simulink model "BANSHEE_v2"  (Simulink 8.1)
settings: Solver=ode1  StartTime=0.0  StopTime=inf  FixedStep=Ts  MaxStep=1e-3  RelTol=1e-3
model workspace (MAT data in the model file):
  op_snapshot1 : opcond.OperatingPoint (value not decoded)
PostLoadFcn:
  | BANSHEE_init;
InitFcn:
  | BANSHEE_init;
values from neighbouring files (symbols this model uses):
  F1 = xlsread('F1_relay_banshee.xlsx')    [relay_settings_init.m]
  F2 = xlsread('F2_relay_banshee.xlsx')    [relay_settings_init.m]
  F3 = xlsread('F3_relay_banshee.xlsx')    [relay_settings_init.m]
  Ts = 100E-6    (= 0.0001)    [BANSHEE_init.m]
undefined symbols (not defined in the file or in its folder): cable_spec, fdesignblkfcn, Feeder1_lib, Feeder2_lib, Feeder3_lib, gcbh, generic_ethernet_cb, Left, relay_housing_lib, SM_UtilityService, SS_F1_RELAY_HOUSING, SS_F2_RELAY_HOUSING, SS_F3_RELAY_HOUSING, SS_Feeder1, SS_Feeder2, SS_Feeder3, type, utility_service_lib, V
libraries: breaker_lib x51, rtio_generic_modbus x43, relay_modbus_lib x42, cables_lib x34, artemis x24, transformer_lib x24, Load_lib x18, simulink x16, ssn_lib x16, rtlab x15, rtio_opalrt_common x15, PQFV_lib x8
(part 1 of 5)
settings Model: ARTEMISmethode_block_infos=$$__separator__$$BANSHEE_v2/ARTEMIS Guide$$__separator__$$  Creator=RE25624  LastModifiedBy=re25624  BufferReuse=off
settings SolverCC: ZeroCrossAlgorithm=Adaptive
settings DataIOCC: ExternalInput=getinputstruct(op_snapshot1)  InitialState=getstatestruct(op_snapshot1)  LimitDataPoints=off  MaxDataPoints=90060  SignalLoggingSaveFormat=Dataset  SaveOutput=off  SignalLogging=off  DSMLogging=off  SaveTime=off  OutputSaveName=result
settings OptimizationCC: BlockReduction=off  OptimizeBlockIOStorage=off  BufferReuse=off  ExpressionFolding=off  LocalBlockOutputs=off
settings DebuggingCC: MaxConsecutiveZCsMsg=warning  IgnoredZcDiagnostic=none  SolverPrmCheckMsg=none  MultiTaskRateTransMsg=warning  FcnCallInpInsideContextMsg=EnableAllAsWarning  FrameProcessingCompatibilityMsg=error  ModelReferenceExtraNoncontSigs=warning  StrictBusMsg=None
settings ModelReferenceCC: UpdateModelReferenceTargets=IfOutOfDate
settings SFSimCC: SFSimEcho=off
settings GRTTargetCC: CodeReplacementLibrary=C89/C90 (ANSI)

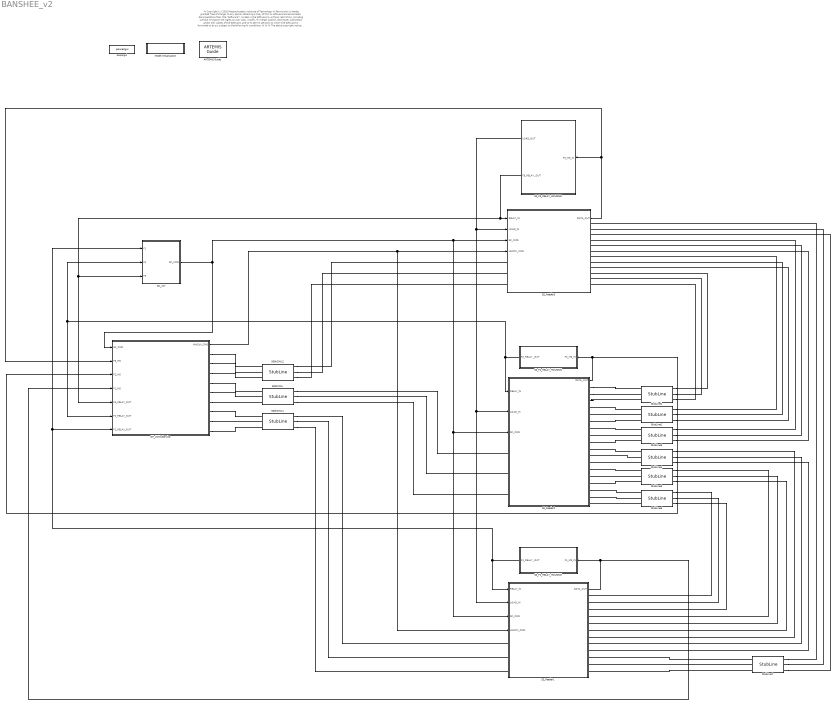
== system BANSHEE_v2 ==
  note: % Copyright (c) 2016 Massachusetts Institute of Technology
      | % Permission is hereby granted, free of charge, to any person obtaining a copy of this
      | % software and associated documentation files (the "Software"), to deal in the Software
      | % without restriction, including without limitation the rights to use, copy, modify,
      | % merge, publish, distribute, sublicense, and/or sell copies of the Software, and to
      | % permit persons to whom the Software is furnished to do so, subject to the following
      | % conditions:
      | %
      | %
      | % The above copyright notice and this permission notice shall be included in
      | % all copies or substantial portions of the Software.
      | %
      | % THE SOFTWARE IS PROVIDED "AS IS", WITHOUT WARRANTY OF ANY KIND, EXPRESS OR IMPLIED,
      | % INCLUDING BUT NOT LIMITED TO THE WARRANTIES OF MERCHANTABILITY, FITNESS FOR A
      | % PARTICULAR PURPOSE AND NONINFRINGEMENT. IN NO EVENT SHALL THE AUTHORS OR COPYRIGHT
      | % HOLDERS BE LIABLE FOR ANY CLAIM, DAMAGES OR OTHER LIABILITY, WHETHER IN AN ACTION
      | % OF CONTRACT, TORT OR OTHERWISE, ARISING FROM, OUT OF OR IN CONNECTION WITH THE
      | % SOFTWARE OR THE USE OR OTHER DEALINGS IN THE SOFTWARE.
      | %
      | %
      | %%
  500kCMIL : artemis/ARTEMIS/StubLine  Phases=3  pu=off  L=10000 * 9.43453e-08 / 1  Lpu=0.08  R=10000 * 2.28409e-5 / 1  Rpu=0.002  S_base=450e6/3  V_base=230e3/sqrt(3)  F_base=60  Ts=Ts
  500kCMIL1 : artemis/ARTEMIS/StubLine  Phases=3  pu=off  L=10000 * 9.43453e-08 / 1  Lpu=0.08  R=10000 * 2.28409e-5 / 1  Rpu=0.002  S_base=450e6/3  V_base=230e3/sqrt(3)  F_base=60  Ts=Ts
  500kCMIL2 : artemis/ARTEMIS/StubLine  Phases=3  pu=off  L=10000 * 9.43453e-08 / 1  Lpu=0.08  R=10000 * 2.28409e-5 / 1  Rpu=0.002  S_base=450e6/3  V_base=230e3/sqrt(3)  F_base=60  Ts=Ts
  ARTEMIS Guide : artemis/ARTEMIS/ARTEMIS Guide  Tag=FTSSmethode_opal_4hx0r99  Description=5.0_z1  lock=on  Ts=Ts  opt=art5  dyna=off  nb_perm=4  RT_fullcomp=off  ssn=on  ssn_itvc=off  ssn_ivic=off  ssn_ext=off  ssn_solver=Art5 with Backward Euler nodal interface  ssn_impulse=off  ssn_quasimpulse=off  ssn_impulse_loop=5  paraExtinctionThy=off  Thy_Impulse=on  dtc=Off  dtc_opt=normal  ao=on  simtype=off  ct_mac=off  lin_mov=off  lsp=[0.001 2]  spike_skip=Disabled  dtc_extra=1  dtc_sws=normal  dtc_pied=0.5  SPSRulesBlock=SPSRules  tre=on  ctmm=off  LF=off  dpl_type=ARTEMiS DPL  rlc_type=off  custom_type=off  para=on  ssn_ImpulseLoopBlockedStateUpdate=5  ssn_mov_iter_number=5  ssn_switch_iter_number=5
  Model Initialization : Subsystem  AncestorBlock=artemis/Tools /Misc/Model Initialization  mask(Model Functions){InitFcnX=BANSHEE_init;, prel=off, posl=on, inif=on, strf=off}
      mask prompts: InitFcnX "Initialisation"; prel "Preload Function"; posl "PostLoad Function"; inif "InitFcn"; strf "StartFcn"
      mask init:
      | currentBlock = gcb;
      | root = bdroot(currentBlock);
      | 
      | if ~strcmp(get_param(root,'BlockDiagramType'),'library')
      |     if prel==1
      |         set_param(root, 'PreLoadFcn', InitFcnX);
      |     else
      |         set_param(root, 'PreLoadFcn', '');
      |     end
      |     if inif==1
      |         set_param(root, 'InitFcn', InitFcnX);
      |     else
      |         set_param(root, 'InitFcn', '');
      |     end
      |     if strf==1
      |         set_param(root, 'StartFcn', InitFcnX);
      |     else
      |         set_param(root, 'StartFcn', '');
      |     end
      |     if posl==1
      |         set_param(root, 'PostLoadFcn', InitFcnX);
      |     else
      |         set_param(root, 'PostLoadFcn', '');
      |     end
      | end
      | 
      | pos = get_param(currentBlock, 'Position');
      | width = pos(3) - pos(1); height = pos(4) - pos(2);
      | txt = [ upper(root) '\n' '- InitFcn. . . . . '  get_param(root, 'InitFcn') ];
      settings: CopyFcn=set_param(gcb,'LinkStatus','inactive')
      mask Display: text(5, height*0.5, txt, 'horizontalAlignment', 'left', 'verticalAlignment', 'middle') ;
  SC_ctrl : Subsystem
  SM_UtilityService : Subsystem  AncestorBlock=utility_service_lib/SM_UtilityService
  SS_F1_RELAY_HOUSING : Subsystem  AncestorBlock=relay_housing_lib/SS_F1_RELAY_HOUSING
  SS_F2_RELAY_HOUSING : Subsystem  AncestorBlock=relay_housing_lib/SS_F2_RELAY_HOUSING
  SS_F3_RELAY_HOUSING : Subsystem  AncestorBlock=relay_housing_lib/SS_F3_RELAY_HOUSING
  SS_Feeder1 : Subsystem  AncestorBlock=Feeder1_lib/SS_Feeder1
  SS_Feeder2 : Subsystem  AncestorBlock=Feeder2_lib/SS_Feeder2
  SS_Feeder3 : Subsystem  AncestorBlock=Feeder3_lib/SS_Feeder3
  StubLine1 : artemis/ARTEMIS/StubLine  Phases=3  pu=off  L=1500 * 9.43453e-08 / 2  Lpu=0.08  R=1500 * 2.28409e-5 / 2  Rpu=0.002  S_base=450e6/3  V_base=230e3/sqrt(3)  F_base=60  Ts=Ts
  StubLine2 : artemis/ARTEMIS/StubLine  Phases=3  pu=off  L=1500 * 9.43453e-08 / 2  Lpu=0.08  R=1500 * 2.28409e-5 / 2  Rpu=0.002  S_base=450e6/3  V_base=230e3/sqrt(3)  F_base=60  Ts=Ts
  StubLine3 : artemis/ARTEMIS/StubLine  Phases=3  pu=off  L=1500 * 9.43453e-08 / 2  Lpu=0.08  R=1500 * 2.28409e-5 / 2  Rpu=0.002  S_base=450e6/3  V_base=230e3/sqrt(3)  F_base=60  Ts=Ts
  StubLine4 : artemis/ARTEMIS/StubLine  Phases=3  pu=off  L=1000 * 9.43453e-08 / 2  Lpu=0.08  R=1000 * 2.28409e-5 / 2  Rpu=0.002  S_base=450e6/3  V_base=230e3/sqrt(3)  F_base=60  Ts=Ts
  StubLine5 : artemis/ARTEMIS/StubLine  Phases=3  pu=off  L=2000 * 9.43453e-08 / 2  Lpu=0.08  R=2000 * 2.28409e-5 / 2  Rpu=0.002  S_base=450e6/3  V_base=230e3/sqrt(3)  F_base=60  Ts=Ts
  StubLine6 : artemis/ARTEMIS/StubLine  Phases=3  pu=off  L=3000 * 9.43453e-08 / 1  Lpu=0.08  R=3000 * 2.28409e-5 / 1  Rpu=0.002  S_base=450e6/3  V_base=230e3/sqrt(3)  F_base=60  Ts=Ts
  StubLine7 : artemis/ARTEMIS/StubLine  Phases=3  pu=off  L=2000 * 9.43453e-08 / 2  Lpu=0.08  R=2000 * 2.28409e-5 / 2  Rpu=0.002  S_base=450e6/3  V_base=230e3/sqrt(3)  F_base=60  Ts=Ts
  powergui : powerlib/powergui  Priority=2  SimulationMode=Discrete  SolverType=Tustin  SampleTime=Ts  frequency=60  SPID=off  DisableSnubberDevices=off  DisableRonSwitches=off  DisableVfSwitches=off  SwTol=0  Interpol=off  DisplayEquations=off  frequencyindice=0  Pbase=100e6  ErrMax=1e-4  Iterations=50  UnitsV=kV  UnitsW=MW  FunctionMessages=off  echomessages=off  HookPort=off  EnableUseOfTLC=off  x0status=blocks  RestoreLinks=warning  ResistiveCurrentMeasurement=off  Frange=logspace(0,3,50)  Ylog=off  Xlog=off  ShowGrid=off  save=off  variable=ZData  structure=0  ZoomFFT=on  StartTime=0.0  cycles=2  DisplayStyle=off  fundamental=60  FreqAxis=off  MaxFrequency=1000  frequencyindicesteady=1  RmsSteady=1  display=off  Ts=0  methode=off
  wires:
  SS_Feeder3/1(DATA_OUT) -> SM_UtilityService/2(F3_MS), SS_F3_RELAY_HOUSING/1(F3_MS_IN)
  SS_F3_RELAY_HOUSING/2(F3_RELAY _OUT) -> SM_UtilityService/5(F3_RELAY_OUT), SC_ctrl/3(F3), SS_Feeder3/1(RELAY_IN)
  SS_F1_RELAY_HOUSING/1(F1_RELAY _OUT) -> SS_Feeder1/1(RELAY_IN), SC_ctrl/1(F1), SM_UtilityService/7(F1_RELAY_OUT)
  SS_F2_RELAY_HOUSING/1(F2_RELAY _OUT) -> SC_ctrl/2(F2), SM_UtilityService/6(F2_RELAY_OUT), SS_Feeder2/1(RELAY_IN)
  SS_Feeder1/1(DATA_OUT) -> SM_UtilityService/4(F1_MS), SS_F1_RELAY_HOUSING/1(F1_MS_IN)
  SS_Feeder2/1(DATA_OUT) -> SM_UtilityService/3(F2_MS), SS_F2_RELAY_HOUSING/1(F2_MS_IN)
  SC_ctrl/1(SC_CMD) -> SM_UtilityService/1(SC_CMD), SS_Feeder1/3(SC_CMD), SS_Feeder2/3(SC_CMD), SS_Feeder3/3(SC_CMD)
  SS_F3_RELAY_HOUSING/1(LOAD_OUT) -> SS_Feeder3/2(LOAD_IN), SS_Feeder1/2(LOAD_IN), SS_Feeder2/2(LOAD_IN)
  SM_UtilityService/1(HWCtrl_CMD) -> SS_Feeder1/4(HWCtrl_CMD), SS_Feeder3/4(HWCtrl_CMD)
  connections:
  SS_Feeder2/RConn2 -- StubLine1/LConn2
  SS_Feeder2/RConn1 -- StubLine1/LConn1
  SS_Feeder2/RConn3 -- StubLine1/LConn3
  StubLine2/LConn2 -- SS_Feeder2/RConn5
  StubLine2/LConn3 -- SS_Feeder2/RConn6
  StubLine2/LConn1 -- SS_Feeder2/RConn4
  StubLine3/LConn2 -- SS_Feeder2/RConn8
  StubLine3/LConn1 -- SS_Feeder2/RConn7
  StubLine3/LConn3 -- SS_Feeder2/RConn9
  StubLine4/LConn3 -- SS_Feeder2/RConn12
  StubLine4/LConn2 -- SS_Feeder2/RConn11
  StubLine4/LConn1 -- SS_Feeder2/RConn10
  StubLine7/LConn3 -- SS_Feeder1/RConn12
  StubLine7/LConn2 -- SS_Feeder1/RConn11
  StubLine7/LConn1 -- SS_Feeder1/RConn10
  StubLine5/LConn2 -- SS_Feeder2/RConn14
  StubLine5/LConn1 -- SS_Feeder2/RConn13
  StubLine5/LConn3 -- SS_Feeder2/RConn15
  StubLine6/LConn3 -- SS_Feeder2/RConn18
  StubLine6/LConn2 -- SS_Feeder2/RConn17
  StubLine6/LConn1 -- SS_Feeder2/RConn16
  StubLine6/RConn1 -- SS_Feeder1/RConn1
  StubLine6/RConn2 -- SS_Feeder1/RConn2
  StubLine6/RConn3 -- SS_Feeder1/RConn3
  StubLine5/RConn1 -- SS_Feeder1/RConn4
  StubLine5/RConn2 -- SS_Feeder1/RConn5
  StubLine5/RConn3 -- SS_Feeder1/RConn6
  StubLine4/RConn1 -- SS_Feeder1/RConn7
  StubLine4/RConn2 -- SS_Feeder1/RConn8
  StubLine4/RConn3 -- SS_Feeder1/RConn9
  StubLine3/RConn3 -- SS_Feeder3/RConn6
  StubLine3/RConn2 -- SS_Feeder3/RConn5
  StubLine3/RConn1 -- SS_Feeder3/RConn4
  StubLine2/RConn3 -- SS_Feeder3/RConn9
  StubLine2/RConn2 -- SS_Feeder3/RConn8
  StubLine2/RConn1 -- SS_Feeder3/RConn7
  StubLine1/RConn3 -- SS_Feeder3/RConn12
  StubLine1/RConn2 -- SS_Feeder3/RConn11
  StubLine1/RConn1 -- SS_Feeder3/RConn10
  StubLine7/RConn1 -- SS_Feeder3/RConn1
  StubLine7/RConn2 -- SS_Feeder3/RConn2
  StubLine7/RConn3 -- SS_Feeder3/RConn3
  500kCMIL2/RConn3 -- SS_Feeder3/LConn3
  500kCMIL2/RConn2 -- SS_Feeder3/LConn2
  500kCMIL2/RConn1 -- SS_Feeder3/LConn1
  500kCMIL/RConn1 -- SS_Feeder2/LConn1
  500kCMIL/RConn2 -- SS_Feeder2/LConn2
  500kCMIL/RConn3 -- SS_Feeder2/LConn3
  500kCMIL1/RConn1 -- SS_Feeder1/LConn1
  500kCMIL1/RConn2 -- SS_Feeder1/LConn2
  500kCMIL1/RConn3 -- SS_Feeder1/LConn3
  SM_UtilityService/RConn1 -- 500kCMIL2/LConn1
  SM_UtilityService/RConn2 -- 500kCMIL2/LConn2
  SM_UtilityService/RConn3 -- 500kCMIL2/LConn3
  SM_UtilityService/RConn4 -- 500kCMIL/LConn1
  SM_UtilityService/RConn5 -- 500kCMIL/LConn2
  SM_UtilityService/RConn6 -- 500kCMIL/LConn3
  SM_UtilityService/RConn7 -- 500kCMIL1/LConn1
  SM_UtilityService/RConn8 -- 500kCMIL1/LConn2
  SM_UtilityService/RConn9 -- 500kCMIL1/LConn3

== system BANSHEE_v2/Model Initialization ==

== system BANSHEE_v2/SC_ctrl ==
  note: % Copyright (c) 2016 Massachusetts Institute of Technology
      | % Permission is hereby granted, free of charge, to any person obtaining a copy of this
      | % software and associated documentation files (the "Software"), to deal in the Software
      | % without restriction, including without limitation the rights to use, copy, modify,
      | % merge, publish, distribute, sublicense, and/or sell copies of the Software, and to
      | % permit persons to whom the Software is furnished to do so, subject to the following
      | % conditions:
      | %
      | %
      | % The above copyright notice and this permission notice shall be included in
      | % all copies or substantial portions of the Software.
      | %
      | % THE SOFTWARE IS PROVIDED "AS IS", WITHOUT WARRANTY OF ANY KIND, EXPRESS OR IMPLIED,
      | % INCLUDING BUT NOT LIMITED TO THE WARRANTIES OF MERCHANTABILITY, FITNESS FOR A
      | % PARTICULAR PURPOSE AND NONINFRINGEMENT. IN NO EVENT SHALL THE AUTHORS OR COPYRIGHT
      | % HOLDERS BE LIABLE FOR ANY CLAIM, DAMAGES OR OTHER LIABILITY, WHETHER IN AN ACTION
      | % OF CONTRACT, TORT OR OTHERWISE, ARISING FROM, OUT OF OR IN CONNECTION WITH THE
      | % SOFTWARE OR THE USE OR OTHER DEALINGS IN THE SOFTWARE.
      | %
      | %
      | %%
  note: The 'Overruns' value should remain at 0.
      | The 'Ttotal' value should be equal to the
      | model Fixed-Step size.
  F1 : Inport
  F2 : Inport  Port=2
  F3 : Inport  Port=3
  1: connect motor 0: disconnect motor : Constant  Value=0
  Bus Creator1 : BusCreator
  Gen_3.5MVA : Subsystem
  OpComm : rtlab/OpComm  nbport=3  groupe_acq=1  subsys_rate=0  st=0  Synchronization=on  Interpolation=on  Threshold=1.0  Missed_Data=off  Sim_Time=off  Samples=off  dynSigOut=off  from_console=0  warning_done=off  writeOpCommFile=off  Offset=off
  Overall : Subsystem
  Status : Subsystem
  Woodward : Subsystem
  opElectricFaultSelector : artemis/Tools /POW faults/opElectricFaultSelector  phase_a=on  phase_b=on  phase_c=on  gnd_fault=on  Tacq=1  Tst=[0.1 0 10]  enable_POW=off  angle_POW=[15 0 10]  Tdr="[0.5 0  10]"  fault_location_menu=No fault  T_init=2
  SC_CMD : Outport
  wires:
  F1/1 -> OpComm/1
  F2/1 -> OpComm/2
  F3/1 -> OpComm/3
  OpComm/1 -> Overall/1(F1), Status/1(F1)
  OpComm/2 -> Status/2(F2), Overall/2(F2)
  OpComm/3 -> Status/3(F3), Overall/3(F3)
  opElectricFaultSelector/1 -> [fault_cmd]
  Bus Creator1/1 -> SC_CMD/1
  1: connect motor 0: disconnect motor/1 -> Bus Creator1/2  "motor_signals"
  [IO_ctrl] -> Bus Creator1/3  "IO ctrl"
  Gen_3.5MVA/1(S) -> Bus Creator1/1  "NGCHP_ManualCtrl"
  Woodward/1(IOctrl) -> [IO_ctrl]
  [fault_cmd] -> Bus Creator1/4  "fault_cmd"

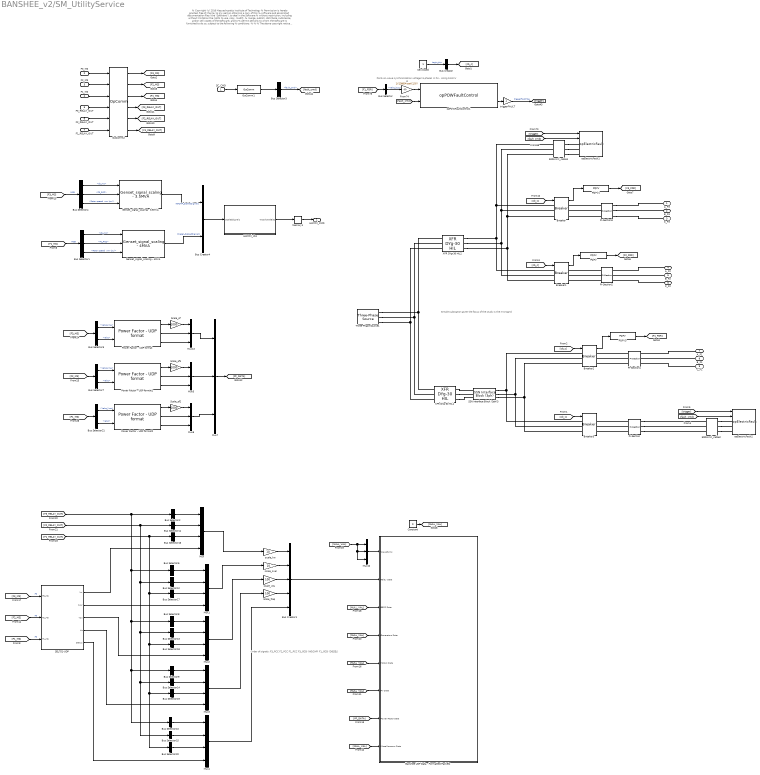
== system BANSHEE_v2/SM_UtilityService ==
  note: Simple substation given the focus of the study is the microgrid
  note: % Copyright (c) 2016 Massachusetts Institute of Technology
      | % Permission is hereby granted, free of charge, to any person obtaining a copy of this
      | % software and associated documentation files (the "Software"), to deal in the Software
      | % without restriction, including without limitation the rights to use, copy, modify,
      | % merge, publish, distribute, sublicense, and/or sell copies of the Software, and to
      | % permit persons to whom the Software is furnished to do so, subject to the following
      | % conditions:
      | %
      | %
      | % The above copyright notice and this permission notice shall be included in
      | % all copies or substantial portions of the Software.
      | %
      | % THE SOFTWARE IS PROVIDED "AS IS", WITHOUT WARRANTY OF ANY KIND, EXPRESS OR IMPLIED,
      | % INCLUDING BUT NOT LIMITED TO THE WARRANTIES OF MERCHANTABILITY, FITNESS FOR A
      | % PARTICULAR PURPOSE AND NONINFRINGEMENT. IN NO EVENT SHALL THE AUTHORS OR COPYRIGHT
      | % HOLDERS BE LIABLE FOR ANY CLAIM, DAMAGES OR OTHER LIABILITY, WHETHER IN AN ACTION
      | % OF CONTRACT, TORT OR OTHERWISE, ARISING FROM, OUT OF OR IN CONNECTION WITH THE
      | % SOFTWARE OR THE USE OR OTHER DEALINGS IN THE SOFTWARE.
      | %
      | %
      | %%
  note: Point-on-wave synchronisation voltage (3-phase) in PU - Using 13.8 kV
  note: Order of signals:
      | F3_PCC
      | F2_PCC
      | F1_PCC
      | F3_GCB (NG/CHP)
      | F1_GCB (DIESEL)
  SC_CMD : Inport
  F3_MS : Inport  Port=2
  F2_MS : Inport  Port=3
  F1_MS : Inport  Port=4
  F3_RELAY_OUT : Inport  Port=5
  F2_RELAY_OUT : Inport  Port=6
  F1_RELAY_OUT : Inport  Port=7
  500kcmil_cable1 : cables_lib/500kcmil_cable  length=1  par_sets=1
  500kcmil_cable2 : cables_lib/500kcmil_cable  length=1  par_sets=1
  Banshee UDP Data - Formatted Packets : Subsystem  mask(UDP Data Block){ProfileID=2, NumOfWaveforms=[0, 0, 0], NumOfRelays=[47, [10, 10, 100, 100]], NumOfBatteries=0, NumOfGensets=0, NumOfMotors=0, NumOfPVs=0, NumOfPF=[3, [1000, 1000, 1000]], NumOfMiscellaneousDataScales=0, NumOfMiscellaneousDataSignalsScales=0}
      mask prompts: ProfileID "Profile ID"; NumOfWaveforms "Waveform Data"; NumOfRelays "Relay Data"; NumOfBatteries "# of Batteries"; NumOfGensets "# of Gensets"; NumOfMotors "# of Motors"; NumOfPVs "# of PVs"; NumOfPF "Power Factor Data"; NumOfMiscellaneousDataScales "Misc. Data - No. of Scale Factors"; NumOfMiscellaneousDataSignalsScales "Misc. - No. Signals and Scale Values"
      mask help:
      | * All signal scaling should be external to this block
      |
      | Profile ID: (1-Sheriff, 2-Banshee, 3-Canary, 4-Siren)
      |
      | Waveforms Data: No. of per phase waveforms sent at 5Hz rate, point per waveforms [dt=80us, 208; dt=100us, 166], and scaling factor.
      | -Input format: [No. of waveforms, No. of datapoints, scale]
      | -Ex. for Canary:[3, 166, 100]
      |
      | Relay Data: No. of relays feeding packet data to breakers in display - mapped/indexed in ascending order
      | -Packet order: Active power(kW), reactive power(kVAR), voltage(per-unit), frequency (Hz), breaker status (1:closed, 0:open)
      | -Input format: [No. of Relays, [scale_kW, scale_kVAR, scale_Vpu, scale_Hz]]
      | -Ex. for Canary:[4, [10, 10, 100, 100]]
      |
      | No. of Batteries: TBD
      | -Ex. for Canary: [0]
      | No. of Generators: TBD
      | -Ex. for Canary: [0]
      |
      | Motors Data: No. of motors monitored in the system. Currently, only looking at motor on/off state.
      | -Input format: [No. of motors]
      | -Ex. for Canary: [1]
      |
      | No. of PV: TBD
      | -Ex. for Canary: [0]
      |
      | Power Factor Data: No. of power factors to be displayed in the system, and corresponding scale values.
      | -Packet order: power factor, import/export, lagging/leading
      | -Input format: [No. of Power Factors, [scale_pf]]
      | -Ex. for Canary:[1, [1000]]
      |
      | Misc. Data - No. of Scale factor: NUmber of scale factors to be applied to each signal-set.
      | -Ex. for Canary: [3]
      |
      | Misc. Data - No. of Signals and Scale Values: Size of signal set and scale value to be applied to the signal-set.
      | -Ex. for Canary: [[1, 1000], [6, 100], [3, 10]]
  Breaker{,1..3} (4 alike) : breaker_lib/Breaker  Ts=Ts  mech_delay=cb_mech_delay
  Bus Creator : BusCreator  Inputs=1
  Bus Creator1 : BusCreator  Inputs=5
  Bus Creator4 : BusCreator  Inputs=2
  Bus Selector : BusSelector  OutputSignals=cb_ms.Vabc_bus
  Bus Selector1 : BusSelector  OutputSignals="DIESEL_DATA.DIESEL_GCB.cb_ms,CB_DATA.F1_PCC,DIESEL_DATA.Gen2_meas.w.w.Rotor speed  wm (pu)"
  Bus Selector10 : BusSelector  OutputSignals=F3_CB_1.m.status,F3_CB_2.m.status,F3_CB_3.m.status,F3_CB_4.m.status,F3_CB_5.m.status,F3_CB_6.m.status,F3_CB_7.m.status,F3_CB_8.m.status,F3_CB_9.m.status  OutputAsBus=on
  Bus Selector11 : BusSelector  OutputSignals=F2_CB_1.m.kw,F2_CB_2.m.kw,F2_CB_3.m.kw,F2_CB_4.m.kw,F2_CB_5.m.kw,F2_CB_6.m.kw,F2_CB_7.m.kw,F2_CB_8.m.kw,F2_CB_9.m.kw,F2_CB_10.m.kw,F2_CB_11.m.kw,F2_CB_12.m.kw,F2_CB_13.m.kw,F2_CB_14.m.kw,F2_CB_15.m.kw,F2_CB_16.m.kw,F2_CB_17.m.kw,F2_CB_18.m.kw,F2_CB_19.m.kw  OutputAsBus=on
  Bus Selector12 : BusSelector  OutputSignals=F2_CB_1.m.kvar,F2_CB_2.m.kvar,F2_CB_3.m.kvar,F2_CB_4.m.kvar,F2_CB_5.m.kvar,F2_CB_6.m.kvar,F2_CB_7.m.kvar,F2_CB_8.m.kvar,F2_CB_9.m.kvar,F2_CB_10.m.kvar,F2_CB_11.m.kvar,F2_CB_12.m.kvar,F2_CB_13.m.kvar,F2_CB_14.m.kvar,F2_CB_15.m.kvar,F2_CB_16.m.kvar,F2_CB_17.m.kvar,F2_CB_18.m.kvar,F2_CB_19.m.kvar  OutputAsBus=on
  Bus Selector13 : BusSelector  OutputSignals=F2_CB_1.m.Vpu,F2_CB_2.m.Vpu,F2_CB_3.m.Vpu,F2_CB_4.m.Vpu,F2_CB_5.m.Vpu,F2_CB_6.m.Vpu,F2_CB_7.m.Vpu,F2_CB_8.m.Vpu,F2_CB_9.m.Vpu,F2_CB_10.m.Vpu,F2_CB_11.m.Vpu,F2_CB_12.m.Vpu,F2_CB_13.m.Vpu,F2_CB_14.m.Vpu,F2_CB_15.m.Vpu,F2_CB_16.m.Vpu,F2_CB_17.m.Vpu,F2_CB_18.m.Vpu,F2_CB_19.m.Vpu  OutputAsBus=on
  Bus Selector14 : BusSelector  OutputSignals=F2_CB_1.m.Hz,F2_CB_2.m.Hz,F2_CB_3.m.Hz,F2_CB_4.m.Hz,F2_CB_5.m.Hz,F2_CB_6.m.Hz,F2_CB_7.m.Hz,F2_CB_8.m.Hz,F2_CB_9.m.Hz,F2_CB_10.m.Hz,F2_CB_11.m.Hz,F2_CB_12.m.Hz,F2_CB_13.m.Hz,F2_CB_14.m.Hz,F2_CB_15.m.Hz,F2_CB_16.m.Hz,F2_CB_17.m.Hz,F2_CB_18.m.Hz,F2_CB_19.m.Hz  OutputAsBus=on
  Bus Selector15 : BusSelector  OutputSignals=F2_CB_1.m.status,F2_CB_2.m.status,F2_CB_3.m.status,F2_CB_4.m.status,F2_CB_5.m.status,F2_CB_6.m.status,F2_CB_7.m.status,F2_CB_8.m.status,F2_CB_9.m.status,F2_CB_10.m.status,F2_CB_11.m.status,F2_CB_12.m.status,F2_CB_13.m.status,F2_CB_14.m.status,F2_CB_15.m.status,F2_CB_16.m.status,F2_CB_17.m.status,F2_CB_18.m.status,F2_CB_19.m.status  OutputAsBus=on
  Bus Selector16 : BusSelector  OutputSignals=F1_CB_1.m.kw,F1_CB_2.m.kw,F1_CB_3.m.kw,F1_CB_4.m.kw,F1_CB_5.m.kw,F1_CB_6.m.kw,F1_CB_7.m.kw,F1_CB_8.m.kw,F1_CB_9.m.kw,F1_CB_10.m.kw,F1_CB_11.m.kw,F1_CB_12.m.kw,F1_CB_13.m.kw,F1_CB_14.m.kw  OutputAsBus=on
  Bus Selector17 : BusSelector  OutputSignals=F1_CB_1.m.kvar,F1_CB_2.m.kvar,F1_CB_3.m.kvar,F1_CB_4.m.kvar,F1_CB_5.m.kvar,F1_CB_6.m.kvar,F1_CB_7.m.kvar,F1_CB_8.m.kvar,F1_CB_9.m.kvar,F1_CB_10.m.kvar,F1_CB_12.m.kvar,F1_CB_11.m.kvar,F1_CB_13.m.kvar,F1_CB_14.m.kvar  OutputAsBus=on
  Bus Selector18 : BusSelector  OutputSignals=F1_CB_1.m.Vpu,F1_CB_2.m.Vpu,F1_CB_3.m.Vpu,F1_CB_4.m.Vpu,F1_CB_5.m.Vpu,F1_CB_6.m.Vpu,F1_CB_7.m.Vpu,F1_CB_8.m.Vpu,F1_CB_9.m.Vpu,F1_CB_10.m.Vpu,F1_CB_11.m.Vpu,F1_CB_12.m.Vpu,F1_CB_13.m.Vpu,F1_CB_14.m.Vpu  OutputAsBus=on
  Bus Selector19 : BusSelector  OutputSignals=F1_CB_1.m.Hz,F1_CB_2.m.Hz,F1_CB_3.m.Hz,F1_CB_4.m.Hz,F1_CB_5.m.Hz,F1_CB_6.m.Hz,F1_CB_7.m.Hz,F1_CB_8.m.Hz,F1_CB_9.m.Hz,F1_CB_10.m.Hz,F1_CB_11.m.Hz,F1_CB_12.m.Hz,F1_CB_13.m.Hz,F1_CB_14.m.Hz  OutputAsBus=on
  Bus Selector2 : BusSelector  OutputSignals=F3_CB_1.m.kw,F3_CB_2.m.kw,F3_CB_3.m.kw,F3_CB_4.m.kw,F3_CB_5.m.kw,F3_CB_6.m.kw,F3_CB_7.m.kw,F3_CB_8.m.kw,F3_CB_9.m.kw  OutputAsBus=on
  Bus Selector20 : BusSelector  OutputSignals=F1_CB_1.m.status,F1_CB_2.m.status,F1_CB_3.m.status,F1_CB_4.m.status,F1_CB_5.m.status,F1_CB_6.m.status,F1_CB_7.m.status,F1_CB_8.m.status,F1_CB_9.m.status,F1_CB_10.m.status,F1_CB_11.m.status,F1_CB_12.m.status,F1_CB_13.m.status,F1_CB_14.m.status  OutputAsBus=on
  Bus Selector21 : BusSelector  OutputSignals=CB_DATA.F1_PCC.Vabc_line,CB_DATA.F1_PCC.Iabc
  Bus Selector3 : BusSelector  OutputSignals=fault_cmd
  Bus Selector4 : BusSelector  OutputSignals="NG_CHP_DATA.NG_CHP_GCB.cb_ms,CB_DATA.F3_PCC,NG_CHP_DATA.Gen1_meas.w.w.Rotor speed  wm (pu)"
  Bus Selector5 : BusSelector  OutputSignals=CB_DATA.F3_PCC.Vabc_line,CB_DATA.F3_PCC.Iabc
  Bus Selector6 : BusSelector  OutputSignals=F3_CB_1.m.kvar,F3_CB_2.m.kvar,F3_CB_3.m.kvar,F3_CB_4.m.kvar,F3_CB_5.m.kvar,F3_CB_6.m.kvar,F3_CB_7.m.kvar,F3_CB_8.m.kvar,F3_CB_9.m.kvar  OutputAsBus=on
  Bus Selector7 : BusSelector  OutputSignals=CB_DATA.F2_PCC.Vabc_line,CB_DATA.F2_PCC.Iabc
  Bus Selector8 : BusSelector  OutputSignals=F3_CB_1.m.Vpu,F3_CB_2.m.Vpu,F3_CB_3.m.Vpu,F3_CB_4.m.Vpu,F3_CB_5.m.Vpu,F3_CB_6.m.Vpu,F3_CB_7.m.Vpu,F3_CB_8.m.Vpu,F3_CB_9.m.Vpu  OutputAsBus=on
  Bus Selector9 : BusSelector  OutputSignals=F3_CB_1.m.Hz,F3_CB_2.m.Hz,F3_CB_3.m.Hz,F3_CB_4.m.Hz,F3_CB_5.m.Hz,F3_CB_6.m.Hz,F3_CB_7.m.Hz,F3_CB_8.m.Hz,F3_CB_9.m.Hz  OutputAsBus=on
  CB closed : Constant
  Constant : Constant  Value=0
  Genset_signal_scaling - 3.5MVA : EasyGen3500_GensetSignalScaling_lib/Genset_signal_scaling - 3.5MVA  Vpk_mcb=11268  watt_mcb=3150000  Vpk_gcb=11268  watt_gcb=3150000  rated_rpm=1800  wm_noise_bias=0.02
  Genset_signal_scaling - 4MVA : EasyGen3500_GensetSignalScaling_lib/Genset_signal_scaling - 4MVA  Vpk_mcb=11268  watt_mcb=3600000  Vpk_gcb=11268  watt_gcb=3600000  rated_rpm=1800  wm_noise_bias=0.02
  HWCtrl_IOs : Subsystem
  Memory1 : Memory
  Mux{,1..4} (5 alike) : Mux
  Mux{5..7,10,13} (5 alike) : Mux  Inputs=3
  OpComm1 : rtlab/OpComm  nbport=1  groupe_acq=1  subsys_rate=0  st=0  Synchronization=on  Interpolation=on  Threshold=1.0  Missed_Data=off  Sim_Time=off  Samples=off  dynSigOut=off  from_console=1  warning_done=off  writeOpCommFile=off  Offset=off
  OpComm2 : rtlab/OpComm  nbport=6  groupe_acq=1  subsys_rate=0  st=0  Synchronization=on  Interpolation=on  Threshold=1.0  Missed_Data=off  Sim_Time=off  Samples=off  dynSigOut=off  from_console=0  warning_done=off  writeOpCommFile=off  Offset=off
  PI-Section : cables_lib/PI-Section  cable_spec=[cable_spec(13, :)]  line_length=3000  parallel_sets=1
  PI-Section1 : cables_lib/PI-Section  cable_spec=[cable_spec(13, :)]  line_length=500  parallel_sets=1
  PI-Section2 : cables_lib/PI-Section  cable_spec=[cable_spec(13, :)]  line_length=500  parallel_sets=1
  PI-Section3 : cables_lib/PI-Section  cable_spec=[cable_spec(13, :)]  line_length=500  parallel_sets=1
  PQFV : PQFV_lib/PQFV  VRMSLL=13800
  PQFV1 : PQFV_lib/PQFV  VRMSLL=13800
  PQFV3 : PQFV_lib/PQFV  VRMSLL=13800
  Power Factor - UDP format : udp_powerfactor_lib/Power Factor - UDP format
  Power Factor - UDP format1 : udp_powerfactor_lib/Power Factor - UDP format
  Power Factor - UDP format2 : udp_powerfactor_lib/Power Factor - UDP format
  SEL751-UDP : Subsystem
  SSN Interface Block (3ph)3 : ssn_lib/SSN Interface Block (3ph)  nb_phase=3  nb_port=2  p1_type=V-type(Left)  p2_type=V-type (Right)  p3_type=V-type(Left)  p4_type=V-type(Left)  p5_type=V-type(Left)  p6_type=V-type(Left)  p7_type=V-type(Left)  p8_type=V-type(Left)  p9_type=V-type(Left)  p10_type=V-type(Left)  p11_type=V-type(Left)  p12_type=V-type(Left)  p13_type=V-type(Left)  p14_type=V-type(Left)  p15_type=V-type(Left)  p16_type=V-type(Left)  I_port_shunt_resistance=1e9
  Scale_freq : Gain  Gain=100
  Scale_pf : Gain  Gain=1000
  Scale_pf1 : Gain  Gain=1000
  Scale_pf2 : Gain  Gain=1000
  Three-Phase Source1 : powerlib/Electrical Sources/Three-Phase Source  Voltage=115000  PhaseAngle=0  Frequency=60  InternalConnection=Yg  SpecifyImpedance=on  Resistance=0.8929  Inductance=16.58e-3  ShortCircuitLevel=100e6  BaseVoltage=115000  XRratio=30  BusType=swing  Pref=0  Qref=0  Qmin=-inf  Qmax=inf
  XFR DYg-30 HIL1 : transformer_lib/XFR DYg-30 HIL  Rating=50000  Vp=115000  Vs=13800  Z=15  XR=30
  XFR DYg-30 HIL2 : transformer_lib/XFR DYg-30 HIL  Rating=50000  Vp=115000  Vs=13800  Z=15  XR=30
  a : Gain  Gain=1/(13800*sqrt(2/3))
  opElectricFault1 : artemis/Tools /POW faults/opElectricFault  FaultLocation=location 7  FaultResistance=0.0001  GroundResistance=0.0001  InitialStates=[0 0 0]  SnubberResistance=1e6  SnubberCapacitance=inf
  opElectricFault2 : artemis/Tools /POW faults/opElectricFault  FaultLocation=location 8  FaultResistance=0.0001  GroundResistance=0.0001  InitialStates=[0 0 0]  SnubberResistance=1e6  SnubberCapacitance=inf
  opPOWFaultControl1 : artemis/Tools /POW faults/opPOWFaultControl  Ts=Ts  usePLL=off  Fgrid=60  PLL_k=[180 3200 1]  vol_sel=1: rising zero-corssing  SyncPhase_menu=A  T_acq=0.8
  scale_kvar : Gain  Gain=10
  scale_kw : Gain  Gain=10
  scale_vpu : Gain  Gain=100
  triggerFAULT : Gain
  A_F3 : PMIOPort  Port=1  Side=Right
  B_F3 : PMIOPort  Port=2  Side=Right
  C_F3 : PMIOPort  Port=3  Side=Right
  A_F2 : PMIOPort  Port=4  Side=Right
  B_F2 : PMIOPort  Port=5  Side=Right
  C_F2 : PMIOPort  Port=6  Side=Right
  A_F1 : PMIOPort  Port=7  Side=Right
  B_F1 : PMIOPort  Port=8  Side=Right
  C_F1 : PMIOPort  Port=9  Side=Right
  HWCtrl_CMD : Outport
  wires:
  [cb_c] -> Breaker2/1
  [cb_c] -> Breaker/1
  [cb_c] -> Breaker1/1
  [cb_c] -> Breaker3/1
  Bus Creator/1 -> [cb_c]
  CB closed/1 -> Bus Creator/1  "Logic_trip"
  [fault_cmd] -> opElectricFault1/2
  [trigger] -> opElectricFault1/1
  [fault_cmd] -> opPOWFaultControl1/2
  opPOWFaultControl1/2 -> triggerFAULT/1
  triggerFAULT/1 -> [trigger]  "triggerFAULTsig"
  [F1_FDR] -> Bus Selector/1
  Bus Selector/1 -> a/1  "<Vabc_bus>"
  a/1 -> opPOWFaultControl1/1
  [fault_cmd] -> opElectricFault2/2
  [trigger] -> opElectricFault2/1
  SC_CMD/1 -> OpComm1/1
  OpComm1/1 -> Bus Selector3/1
  Bus Selector3/1 -> [fault_cmd]  "<fault_cmd>"
  Memory1/1 -> HWCtrl_CMD/1
  Genset_signal_scaling - 3.5MVA/1 -> Bus Creator4/1  "NGCHP_ScaledSignals"
  Genset_signal_scaling - 4MVA/1 -> Bus Creator4/2  "Diesel_ScaledSignals"
  [F3_MS] -> Bus Selector4/1  "MCB"
  Bus Selector4/3 -> Genset_signal_scaling - 3.5MVA/3  "<Rotor speed  wm (pu)>"
  Bus Selector4/2 -> Genset_signal_scaling - 3.5MVA/2  "<F3_PCC>"
  Bus Selector4/1 -> Genset_signal_scaling - 3.5MVA/1  "<cb_ms>"
  Bus Creator4/1 -> HWCtrl_IOs/1(ScaledSignals)
  HWCtrl_IOs/1(WoodwardBias) -> Memory1/1
  [F1_MS] -> Bus Selector1/1  "MCB"
  Bus Selector1/3 -> Genset_signal_scaling - 4MVA/3  "<Rotor speed  wm (pu)>"
  Bus Selector1/2 -> Genset_signal_scaling - 4MVA/2  "<F1_PCC>"
  Bus Selector1/1 -> Genset_signal_scaling - 4MVA/1  "<cb_ms>"
  F2_MS/1 -> OpComm2/2
  F1_MS/1 -> OpComm2/3
  F3_MS/1 -> OpComm2/1
  OpComm2/1 -> [F3_MS]
  OpComm2/2 -> [F2_MS]
  OpComm2/3 -> [F1_MS]
  Breaker/1 -> PQFV1/1
  Breaker1/1 -> PQFV/1
  Breaker2/1 -> PQFV3/1
  PQFV3/1 -> [F1_FDR]
  PQFV1/1 -> [F3_FDR]
  PQFV/1 -> [F2_FDR]
  [F3_MS] -> SEL751-UDP/1(F3_MS)  "F3"
  [F2_MS] -> SEL751-UDP/2(F2_MS)  "F3"
  [F1_MS] -> SEL751-UDP/3(F1_MS)  "F3"
  [NULL_VAL] -> Mux10/1, Mux10/2, Mux10/3
  Mux10/1 -> Banshee UDP Data - Formatted Packets/1(Waveforms)
  Constant/1 -> [NULL_VAL]
  Bus Creator1/1 -> Banshee UDP Data - Formatted Packets/2(Relay Data)
  scale_kw/1 -> Bus Creator1/1
  scale_kvar/1 -> Bus Creator1/2
  Scale_freq/1 -> Bus Creator1/4
  scale_vpu/1 -> Bus Creator1/3
  Mux/1 -> scale_kw/1
  Mux1/1 -> scale_kvar/1
  Mux2/1 -> scale_vpu/1
  Mux3/1 -> Scale_freq/1
  Mux4/1 -> Bus Creator1/5
  [NULL_VAL] -> Banshee UDP Data - Formatted Packets/4(Generators Data)
  [NULL_VAL] -> Banshee UDP Data - Formatted Packets/3(BESS Data)
  [NULL_VAL] -> Banshee UDP Data - Formatted Packets/5(Motors Data)
  [NULL_VAL] -> Banshee UDP Data - Formatted Packets/6(PV Data)
  [NULL_VAL] -> Banshee UDP Data - Formatted Packets/8(Miscellaneous Data)
  [PF_DATA] -> Banshee UDP Data - Formatted Packets/7(Power Factor Data)
  Bus Selector2/1 -> Mux/1
  Bus Selector6/1 -> Mux1/1
  Bus Selector8/1 -> Mux2/1
  Bus Selector9/1 -> Mux3/1
  Bus Selector10/1 -> Mux4/1
  [F3_RELAY_OUT] -> Bus Selector2/1, Bus Selector6/1, Bus Selector8/1, Bus Selector9/1, Bus Selector10/1
  Bus Selector12/1 -> Mux1/2
  Bus Selector11/1 -> Mux/2
  Bus Selector13/1 -> Mux2/2
  Bus Selector15/1 -> Mux4/2
  Bus Selector14/1 -> Mux3/2
  [F2_RELAY_OUT] -> Bus Selector11/1, Bus Selector12/1, Bus Selector13/1, Bus Selector14/1, Bus Selector15/1
  Bus Selector20/1 -> Mux4/3
  Bus Selector19/1 -> Mux3/3
  Bus Selector18/1 -> Mux2/3
  Bus Selector17/1 -> Mux1/3
  Bus Selector16/1 -> Mux/3
  [F1_RELAY_OUT] -> Bus Selector16/1, Bus Selector19/1, Bus Selector20/1, Bus Selector18/1, Bus Selector17/1
  SEL751-UDP/1(kw) -> Mux/4
  SEL751-UDP/2(kvar) -> Mux1/4
  SEL751-UDP/3(Vpu) -> Mux2/4
  SEL751-UDP/4(Hz) -> Mux3/4
  SEL751-UDP/5(Status) -> Mux4/4
  F3_RELAY_OUT/1 -> OpComm2/4
  F1_RELAY_OUT/1 -> OpComm2/6
  F2_RELAY_OUT/1 -> OpComm2/5
  OpComm2/4 -> [F3_RELAY_OUT]
  OpComm2/6 -> [F1_RELAY_OUT]
  OpComm2/5 -> [F2_RELAY_OUT]
  Power Factor - UDP format/1 -> Scale_pf/1
  Scale_pf/1 -> Mux13/1
  [F3_MS] -> Bus Selector5/1
  Bus Selector5/1 -> Power Factor - UDP format/1  "<Vabc_line>"
  Bus Selector5/2 -> Power Factor - UDP format/2  "<Iabc>"
  Power Factor - UDP format/2 -> Mux13/2
  Power Factor - UDP format/3 -> Mux13/3
  Mux13/1 -> Mux7/1
  Power Factor - UDP format1/1 -> Scale_pf1/1
  Scale_pf1/1 -> Mux5/1
  [F2_MS] -> Bus Selector7/1
  Bus Selector7/1 -> Power Factor - UDP format1/1  "<Vabc_line>"
  Bus Selector7/2 -> Power Factor - UDP format1/2  "<Iabc>"
  Power Factor - UDP format1/2 -> Mux5/2
  Power Factor - UDP format1/3 -> Mux5/3
  Mux5/1 -> Mux7/2
  Power Factor - UDP format2/1 -> Scale_pf2/1
  Scale_pf2/1 -> Mux6/1
  [F1_MS] -> Bus Selector21/1
  Bus Selector21/1 -> Power Factor - UDP format2/1  "<Vabc_line>"
  Bus Selector21/2 -> Power Factor - UDP format2/2  "<Iabc>"
  Power Factor - UDP format2/2 -> Mux6/2
  Power Factor - UDP format2/3 -> Mux6/3
  Mux6/1 -> Mux7/3
  Mux7/1 -> [PF_DATA]
  connections:
  PI-Section2/LConn1 -- Breaker1/RConn1
  PI-Section2/LConn3 -- Breaker1/RConn3
  PI-Section1/LConn1 -- Breaker2/RConn1
  PI-Section1/LConn2 -- Breaker2/RConn2
  PI-Section3/LConn1 -- Breaker/RConn1
  PI-Section1/LConn3 -- Breaker2/RConn3
  Breaker3/LConn2 -- SSN Interface Block (3ph)3/RConn2 -- Breaker2/LConn2
  PI-Section3/LConn2 -- Breaker/RConn2
  Breaker3/LConn3 -- SSN Interface Block (3ph)3/RConn3 -- Breaker2/LConn3
  PI-Section/LConn3 -- Breaker3/RConn3
  PI-Section2/LConn2 -- Breaker1/RConn2
  PI-Section/LConn1 -- Breaker3/RConn1
  Breaker3/LConn1 -- SSN Interface Block (3ph)3/RConn1 -- Breaker2/LConn1
  PI-Section3/LConn3 -- Breaker/RConn3
  Breaker1/LConn2 -- 500kcmil_cable1/LConn2 -- Breaker/LConn2 -- XFR DYg-30 HIL2/RConn2
  XFR DYg-30 HIL2/RConn1 -- Breaker1/LConn1 -- 500kcmil_cable1/LConn1 -- Breaker/LConn1
  Breaker1/LConn3 -- 500kcmil_cable1/LConn3 -- Breaker/LConn3 -- XFR DYg-30 HIL2/RConn3
  PI-Section/LConn2 -- Breaker3/RConn2
  A_F2/RConn1 -- PI-Section2/RConn1
  B_F1/RConn1 -- PI-Section1/RConn2
  PI-Section3/RConn3 -- C_F3/RConn1
  Three-Phase Source1/RConn3 -- XFR DYg-30 HIL2/LConn3 -- XFR DYg-30 HIL1/LConn3
  Three-Phase Source1/RConn2 -- XFR DYg-30 HIL2/LConn2 -- XFR DYg-30 HIL1/LConn2
  Three-Phase Source1/RConn1 -- XFR DYg-30 HIL2/LConn1 -- XFR DYg-30 HIL1/LConn1
  C_F2/RConn1 -- PI-Section2/RConn3
  PI-Section3/RConn1 -- A_F3/RConn1
  B_F2/RConn1 -- PI-Section2/RConn2
  A_F1/RConn1 -- PI-Section1/RConn1
  C_F1/RConn1 -- PI-Section1/RConn3
  PI-Section3/RConn2 -- B_F3/RConn1
  500kcmil_cable1/RConn3 -- opElectricFault1/LConn3
  500kcmil_cable1/RConn2 -- opElectricFault1/LConn2
  500kcmil_cable1/RConn1 -- opElectricFault1/LConn1
  500kcmil_cable2/RConn3 -- opElectricFault2/LConn3
  500kcmil_cable2/RConn2 -- opElectricFault2/LConn2
  500kcmil_cable2/RConn1 -- opElectricFault2/LConn1
  PI-Section/RConn3 -- 500kcmil_cable2/LConn3
  PI-Section/RConn2 -- 500kcmil_cable2/LConn2
  PI-Section/RConn1 -- 500kcmil_cable2/LConn1
  XFR DYg-30 HIL1/RConn3 -- SSN Interface Block (3ph)3/LConn3
  XFR DYg-30 HIL1/RConn2 -- SSN Interface Block (3ph)3/LConn2
  XFR DYg-30 HIL1/RConn1 -- SSN Interface Block (3ph)3/LConn1

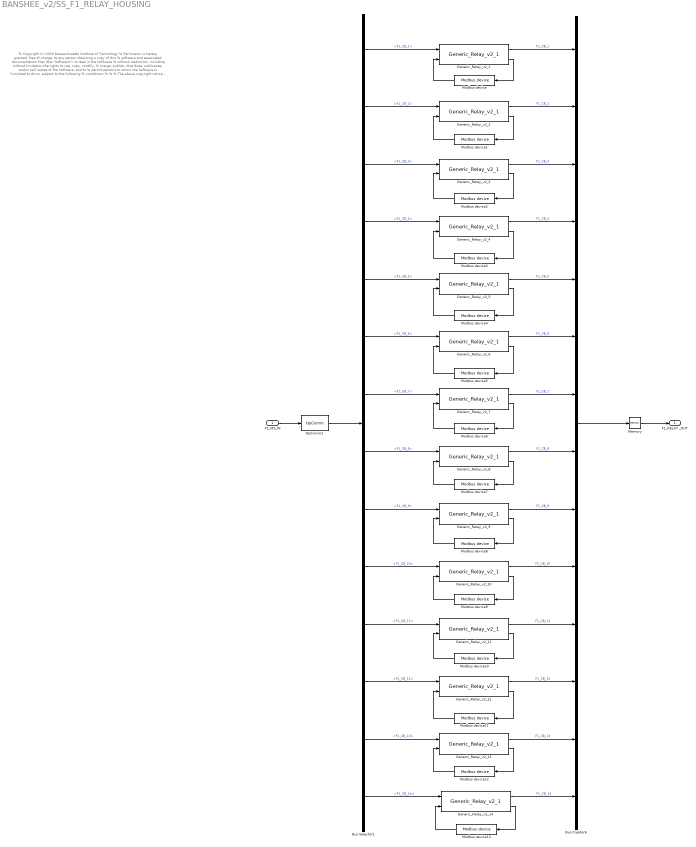
== system BANSHEE_v2/SS_F1_RELAY_HOUSING ==
  note: % Copyright (c) 2016 Massachusetts Institute of Technology
      | % Permission is hereby granted, free of charge, to any person obtaining a copy of this
      | % software and associated documentation files (the "Software"), to deal in the Software
      | % without restriction, including without limitation the rights to use, copy, modify,
      | % merge, publish, distribute, sublicense, and/or sell copies of the Software, and to
      | % permit persons to whom the Software is furnished to do so, subject to the following
      | % conditions:
      | %
      | %
      | % The above copyright notice and this permission notice shall be included in
      | % all copies or substantial portions of the Software.
      | %
      | % THE SOFTWARE IS PROVIDED "AS IS", WITHOUT WARRANTY OF ANY KIND, EXPRESS OR IMPLIED,
      | % INCLUDING BUT NOT LIMITED TO THE WARRANTIES OF MERCHANTABILITY, FITNESS FOR A
      | % PARTICULAR PURPOSE AND NONINFRINGEMENT. IN NO EVENT SHALL THE AUTHORS OR COPYRIGHT
      | % HOLDERS BE LIABLE FOR ANY CLAIM, DAMAGES OR OTHER LIABILITY, WHETHER IN AN ACTION
      | % OF CONTRACT, TORT OR OTHERWISE, ARISING FROM, OUT OF OR IN CONNECTION WITH THE
      | % SOFTWARE OR THE USE OR OTHER DEALINGS IN THE SOFTWARE.
      | %
      | %
      | %%
  F1_MS_IN : Inport
  Bus Creator6 : BusCreator  Inputs=14
  Bus Selector1 : BusSelector  OutputSignals=CB_DATA.F1_CB_1,CB_DATA.F1_CB_2,CB_DATA.F1_CB_3,CB_DATA.F1_CB_4,CB_DATA.F1_CB_5,CB_DATA.F1_CB_6,CB_DATA.F1_CB_7,CB_DATA.F1_CB_8,CB_DATA.F1_CB_9,CB_DATA.F1_CB_10,CB_DATA.F1_CB_11,CB_DATA.F1_CB_12,CB_DATA.F1_CB_13,CB_DATA.F1_CB_14
  Generic_Relay_v2_1 : relay_modbus_lib/Generic_Relay_v2_1  Ts=Ts  relay_settings=[F1(1,:)]
  Generic_Relay_v2_10 : relay_modbus_lib/Generic_Relay_v2_1  Ts=Ts  relay_settings=[F1(10,:)]
  Generic_Relay_v2_11 : relay_modbus_lib/Generic_Relay_v2_1  Ts=Ts  relay_settings=[F1(11,:)]
  Generic_Relay_v2_12 : relay_modbus_lib/Generic_Relay_v2_1  Ts=Ts  relay_settings=[F1(12,:)]
  Generic_Relay_v2_13 : relay_modbus_lib/Generic_Relay_v2_1  Ts=Ts  relay_settings=[F1(13,:)]
  Generic_Relay_v2_14 : relay_modbus_lib/Generic_Relay_v2_1  Ts=Ts  relay_settings=[F1(14,:)]
  Generic_Relay_v2_2 : relay_modbus_lib/Generic_Relay_v2_1  Ts=Ts  relay_settings=[F1(2,:)]
  Generic_Relay_v2_3 : relay_modbus_lib/Generic_Relay_v2_1  Ts=Ts  relay_settings=[F1(3,:)]
  Generic_Relay_v2_4 : relay_modbus_lib/Generic_Relay_v2_1  Ts=Ts  relay_settings=[F1(4,:)]
  Generic_Relay_v2_5 : relay_modbus_lib/Generic_Relay_v2_1  Ts=Ts  relay_settings=[F1(5,:)]
  Generic_Relay_v2_6 : relay_modbus_lib/Generic_Relay_v2_1  Ts=Ts  relay_settings=[F1(6,:)]
  Generic_Relay_v2_7 : relay_modbus_lib/Generic_Relay_v2_1  Ts=Ts  relay_settings=[F1(7,:)]
  Generic_Relay_v2_8 : relay_modbus_lib/Generic_Relay_v2_1  Ts=Ts  relay_settings=[F1(8,:)]
  Generic_Relay_v2_9 : relay_modbus_lib/Generic_Relay_v2_1  Ts=Ts  relay_settings=[F1(9,:)]
  Memory : Memory
  Modbus device : rtio_generic_modbus/Modbus device  conf_name=F1_relay_cfg1.opal  conf_name_mask=F1_relay_cfg1.xls  sample_time=Ts
  Modbus device1 : rtio_generic_modbus/Modbus device  conf_name=F1_relay_cfg2.opal  conf_name_mask=F1_relay_cfg2.xls  sample_time=Ts
  Modbus device10 : rtio_generic_modbus/Modbus device  conf_name=F1_relay_cfg11.opal  conf_name_mask=F1_relay_cfg11.xls  sample_time=Ts
  Modbus device11 : rtio_generic_modbus/Modbus device  conf_name=F1_relay_cfg12.opal  conf_name_mask=F1_relay_cfg12.xls  sample_time=Ts
  Modbus device12 : rtio_generic_modbus/Modbus device  conf_name=F1_relay_cfg13.opal  conf_name_mask=F1_relay_cfg13.xls  sample_time=Ts
  Modbus device13 : rtio_generic_modbus/Modbus device  conf_name=F1_relay_cfg14.opal  conf_name_mask=F1_relay_cfg14.xls  sample_time=Ts
  Modbus device2 : rtio_generic_modbus/Modbus device  conf_name=F1_relay_cfg3.opal  conf_name_mask=F1_relay_cfg3.xls  sample_time=Ts
  Modbus device3 : rtio_generic_modbus/Modbus device  conf_name=F1_relay_cfg4.opal  conf_name_mask=F1_relay_cfg4.xls  sample_time=Ts
  Modbus device4 : rtio_generic_modbus/Modbus device  conf_name=F1_relay_cfg5.opal  conf_name_mask=F1_relay_cfg5.xls  sample_time=Ts
  Modbus device5 : rtio_generic_modbus/Modbus device  conf_name=F1_relay_cfg6.opal  conf_name_mask=F1_relay_cfg6.xls  sample_time=Ts
  Modbus device6 : rtio_generic_modbus/Modbus device  conf_name=F1_relay_cfg7.opal  conf_name_mask=F1_relay_cfg7.xls  sample_time=Ts
  Modbus device7 : rtio_generic_modbus/Modbus device  conf_name=F1_relay_cfg8.opal  conf_name_mask=F1_relay_cfg8.xls  sample_time=Ts
  Modbus device8 : rtio_generic_modbus/Modbus device  conf_name=F1_relay_cfg9.opal  conf_name_mask=F1_relay_cfg9.xls  sample_time=Ts
  Modbus device9 : rtio_generic_modbus/Modbus device  conf_name=F1_relay_cfg10.opal  conf_name_mask=F1_relay_cfg10.xls  sample_time=Ts
  OpComm2 : rtlab/OpComm  nbport=1  groupe_acq=1  subsys_rate=0  st=0  Synchronization=on  Interpolation=on  Threshold=1.0  Missed_Data=off  Sim_Time=off  Samples=off  dynSigOut=off  from_console=0  warning_done=off  writeOpCommFile=off  Offset=off
  F1_RELAY _OUT : Outport
  wires:
  OpComm2/1 -> Bus Selector1/1
  Modbus device12/1 -> Generic_Relay_v2_13/2
  Generic_Relay_v2_13/2 -> Modbus device12/1
  Modbus device11/1 -> Generic_Relay_v2_12/2
  Generic_Relay_v2_12/2 -> Modbus device11/1
  Modbus device10/1 -> Generic_Relay_v2_11/2
  Generic_Relay_v2_11/2 -> Modbus device10/1
  Modbus device9/1 -> Generic_Relay_v2_10/2
  Generic_Relay_v2_10/2 -> Modbus device9/1
  Modbus device8/1 -> Generic_Relay_v2_9/2
  Generic_Relay_v2_9/2 -> Modbus device8/1
  Modbus device7/1 -> Generic_Relay_v2_8/2
  Generic_Relay_v2_8/2 -> Modbus device7/1
  Modbus device6/1 -> Generic_Relay_v2_7/2
  Generic_Relay_v2_7/2 -> Modbus device6/1
  Modbus device5/1 -> Generic_Relay_v2_6/2
  Generic_Relay_v2_6/2 -> Modbus device5/1
  Modbus device4/1 -> Generic_Relay_v2_5/2
  Generic_Relay_v2_5/2 -> Modbus device4/1
  Modbus device3/1 -> Generic_Relay_v2_4/2
  Generic_Relay_v2_4/2 -> Modbus device3/1
  Modbus device2/1 -> Generic_Relay_v2_3/2
  Generic_Relay_v2_3/2 -> Modbus device2/1
  Generic_Relay_v2_2/2 -> Modbus device1/1
  Modbus device1/1 -> Generic_Relay_v2_2/2
  Generic_Relay_v2_1/2 -> Modbus device/1
  Modbus device/1 -> Generic_Relay_v2_1/2
  F1_MS_IN/1 -> OpComm2/1
  Bus Selector1/1 -> Generic_Relay_v2_1/1  "<F1_CB_1>"
  Generic_Relay_v2_1/1 -> Bus Creator6/1  "F1_CB_1"
  Bus Creator6/1 -> Memory/1
  Bus Selector1/2 -> Generic_Relay_v2_2/1  "<F1_CB_2>"
  Generic_Relay_v2_2/1 -> Bus Creator6/2  "F1_CB_2"
  Bus Selector1/3 -> Generic_Relay_v2_3/1  "<F1_CB_3>"
  Bus Selector1/4 -> Generic_Relay_v2_4/1  "<F1_CB_4>"
  Bus Selector1/5 -> Generic_Relay_v2_5/1  "<F1_CB_5>"
  Bus Selector1/6 -> Generic_Relay_v2_6/1  "<F1_CB_6>"
  Bus Selector1/7 -> Generic_Relay_v2_7/1  "<F1_CB_7>"
  Bus Selector1/8 -> Generic_Relay_v2_8/1  "<F1_CB_8>"
  Bus Selector1/9 -> Generic_Relay_v2_9/1  "<F1_CB_9>"
  Bus Selector1/10 -> Generic_Relay_v2_10/1  "<F1_CB_10>"
  Bus Selector1/11 -> Generic_Relay_v2_11/1  "<F1_CB_11>"
  Bus Selector1/12 -> Generic_Relay_v2_12/1  "<F1_CB_12>"
  Bus Selector1/13 -> Generic_Relay_v2_13/1  "<F1_CB_13>"
  Generic_Relay_v2_13/1 -> Bus Creator6/13  "F1_CB_13"
  Generic_Relay_v2_12/1 -> Bus Creator6/12  "F1_CB_12"
  Generic_Relay_v2_11/1 -> Bus Creator6/11  "F1_CB_11"
  Generic_Relay_v2_10/1 -> Bus Creator6/10  "F1_CB_10"
  Generic_Relay_v2_9/1 -> Bus Creator6/9  "F1_CB_9"
  Generic_Relay_v2_8/1 -> Bus Creator6/8  "F1_CB_8"
  Generic_Relay_v2_7/1 -> Bus Creator6/7  "F1_CB_7"
  Generic_Relay_v2_6/1 -> Bus Creator6/6  "F1_CB_6"
  Generic_Relay_v2_5/1 -> Bus Creator6/5  "F1_CB_5"
  Generic_Relay_v2_4/1 -> Bus Creator6/4  "F1_CB_4"
  Generic_Relay_v2_3/1 -> Bus Creator6/3  "F1_CB_3"
  Modbus device13/1 -> Generic_Relay_v2_14/2
  Generic_Relay_v2_14/2 -> Modbus device13/1
  Generic_Relay_v2_14/1 -> Bus Creator6/14  "F1_CB_14"
  Bus Selector1/14 -> Generic_Relay_v2_14/1  "<F1_CB_14>"
  Memory/1 -> F1_RELAY _OUT/1
